simulink library "sensorLibrary"  (R2015b)
settings: Solver=VariableStepAuto  StartTime=0.0  StopTime=10.0  RelTol=1e-3
libraries: frdmkl25zlib x1
settings Model: Creator=dc315  LastModifiedBy=dc315

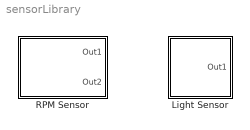
== system sensorLibrary ==
  Light Sensor : Subsystem
      mask Display:
      | pic = imread('light_icon.png');
      | pos = get_param(gcb, 'Position');
      | width  = pos(3) - pos(1);
      | height = pos(4) - pos(2);
      | x = width/2  - 20;
      | y = height/2 - 20;
      | image(pic,[x y 40 40]);
  RPM Sensor : Subsystem
      mask Display:
      | pic = imread('wheel_icon.jpg');
      | pos = get_param(gcb, 'Position');
      | height = pos(4) - pos(2);
      | y = height/2 - 20;
      | image(pic,[10 y 40 40]);
      | port_label('output',1,'left');
      | port_label('output',2,'right');

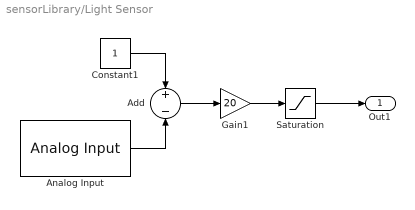
== system sensorLibrary/Light Sensor ==
  Add : Sum  Inputs=+-  AccumDataTypeStr=double  OutDataTypeStr=double
  Analog Input : frdmkl25zlib/Analog Input  WhichPin=A5  SampleTime=0.01
  Constant1 : Constant
  Gain1 : Gain  Gain=20
  Saturation : Saturate  UpperLimit=1  LowerLimit=0  OutDataTypeStr=double
  Out1 : Outport
  wires:
  Add/1 -> Gain1/1
  Analog Input/1 -> Add/2
  Constant1/1 -> Add/1
  Gain1/1 -> Saturation/1
  Saturation/1 -> Out1/1

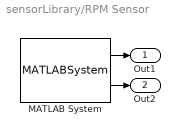
== system sensorLibrary/RPM Sensor ==
  MATLAB System : MATLABSystem  System=freedomboard.rpmSensor  SimulateUsing=Code generation
      mask Type: freedomboard.rpmSensor
      mask Display:
      | disp('rpmSensor');
      | port_label('output',1,'leftRpm');
      | port_label('output',2,'rightRpm');
  Out1 : Outport
  Out2 : Outport  Port=2
  wires:
  MATLAB System/1 -> Out1/1
  MATLAB System/2 -> Out2/1
